simulink library "lib_fuel_cell2"  (Simulink 5.1)
values from neighbouring files (symbols this model uses):
  logFlag = 1    [advSACompMaskInit.m]    (also in advSACompMaskInitR13.m)
undefined symbols (not defined in the file or in its folder): fc_acc_mass, fc_base_mass, fc_c2i_th_cond, fc_c_init_tmp, fc_cl2h_eff, fc_co_map, fc_co_map_c2h, fc_cold, fc_cold_tmp, fc_cp, fc_eff_scale, fc_emisv, fc_exflow_map, fc_ext_sarea, fc_extmp_map, fc_fuel_den, fc_fuel_lhv, fc_fuel_map, fc_fuel_map_c2h, fc_h2x_th_cond, fc_h_air_flow, fc_h_cp, fc_hc_map, fc_hc_map_c2h, fc_hood_emisv, fc_hood_sarea, fc_i2x_th_cond, fc_i_init_tmp, fc_nox_map, fc_nox_map_c2h, fc_o2_map, fc_pm_map, fc_pm_map_c2h, fc_pwr_map, fc_pwr_scale, fc_tstat, pow
libraries: lib_etc x1
(part 2 of 2)

== system lib_fuel_cell2/fuel converter <fc> net model/Subsystem/Subsystem/fuel cell  system <fc>/Block NOTES ==
  note: 7/30/98
      | - started with battery from BD_SER2h.m
      | - added a Saturation block to prevent computed
      |        SOC from falling below 0 or rising above 1
      | - added logic in 'limit power' to prevent discharge
      | if SOC is below 0.001 (0.1%)
      | -added limit block to check if low SOC is preventing
      | discharge
  note: Power loss is computed as I*R+losses due to Coulombic (in)efficiency.
  note: This block models the energy storage system as an SOC-dependent voltage
      | in series with an SOC- and current direction-dependent internal resistance.
      | SOC is computed assuming that A-h capacity is a function of average discharge
      | current:  (A-h capacity)=ess_peukert_coeff * (average discharge current)^ess_peukert_exp.
      |
      | Discharge power is limited here so as not to bring the bus (battery pack) voltage below
      | the minimum controller voltage and so as to allow the solution of the quadratic eq'n for
      | discharge current.
      |
      | Positive current is discharge current in the convention used here.

== system lib_fuel_cell2/fuel converter <fc> net model/Subsystem/Subsystem/fuel cell  system <fc>/pwr vs. eff  fuel cell model ==
  net pwr req (W) : Inport
  Enable : EnablePort  StatesWhenEnabling=reset
  enforce limits : Subsystem
  net pwr avail (W) : Outport  OutputWhenDisabled=reset  InitialOutput=0
  wires:
  enforce limits/1(Out1) -> net pwr avail (W)/1
  net pwr req (W)/1 -> enforce limits/1(In1)

== system lib_fuel_cell2/fuel converter <fc> net model/Subsystem/Subsystem/fuel use and EO emis Fuel Cell/Block NOTES ==
  note: This block determines actual fuel use and engine-out emissions
      | given the fully hot values and the engine coolant temperature.
      | The correlations used here were developed at NREL using
      | FTP data collected under subcontract by JDM & Associates.
      | Note: PM hot/cold relation assumed same as HC

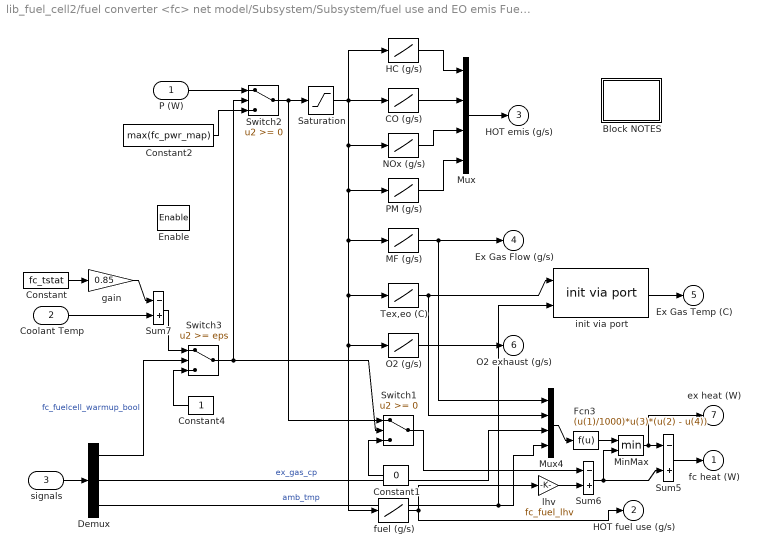
== system lib_fuel_cell2/fuel converter <fc> net model/Subsystem/Subsystem/fuel use and EO emis Fuel Cell/HOT engine maps  ==
  P (W) : Inport
  Coolant Temp : Inport  Port=2
  signals : Inport  Port=3
  Enable : EnablePort  StatesWhenEnabling=reset
  Block NOTES : Subsystem
      mask Display: disp('Block\nNOTES')
  CO (g/s) : Lookup  InputValues=fc_pwr_map*fc_pwr_scale  OutputValues=fc_co_map*fc_pwr_scale  SaturateOnIntegerOverflow=on
  Constant : Constant  Value=fc_tstat
  Constant1 : Constant  Orientation=left  Value=0
  Constant2 : Constant  Value=max(fc_pwr_map)
  Constant4 : Constant  Orientation=left
  Demux : Demux  Outputs=3
  Fcn3 : Fcn  Expr=(u(1)/1000)*u(3)*(u(2) - u(4))
  HC (g/s) : Lookup  InputValues=fc_pwr_map*fc_pwr_scale  OutputValues=fc_hc_map*fc_pwr_scale  SaturateOnIntegerOverflow=on
  MF (g/s) : Lookup  InputValues=fc_pwr_map*fc_pwr_scale  OutputValues=fc_exflow_map*fc_pwr_scale  SaturateOnIntegerOverflow=on
  MinMax : MinMax  Inputs=2
  Mux : Mux
  Mux4 : Mux
  NOx (g/s) : Lookup  InputValues=fc_pwr_map*fc_pwr_scale  OutputValues=fc_nox_map*fc_pwr_scale  SaturateOnIntegerOverflow=on
  O2 (g/s) : Lookup  InputValues=fc_pwr_map*fc_pwr_scale  OutputValues=fc_o2_map*fc_pwr_scale  SaturateOnIntegerOverflow=on
  PM (g/s) : Lookup  InputValues=fc_pwr_map*fc_pwr_scale  OutputValues=fc_pm_map*fc_pwr_scale  SaturateOnIntegerOverflow=on
  Saturation : Saturate  UpperLimit=max(fc_pwr_map*fc_pwr_scale)  LowerLimit=0
  Sum5 : Sum  Inputs=-+  SaturateOnIntegerOverflow=on  InputSameDT=on
  Sum6 : Sum  Inputs=-+  SaturateOnIntegerOverflow=on  InputSameDT=on
  Sum7 : Sum  Inputs=-+  SaturateOnIntegerOverflow=on  InputSameDT=on
  Switch1 : Switch  SaturateOnIntegerOverflow=on  InputSameDT=on
  Switch2 : Switch  SaturateOnIntegerOverflow=on  InputSameDT=on
  Switch3 : Switch  Threshold=eps  SaturateOnIntegerOverflow=on  InputSameDT=on
  Tex,eo (C) : Lookup  InputValues=fc_pwr_map*fc_pwr_scale  OutputValues=fc_extmp_map  SaturateOnIntegerOverflow=on
  fuel (g/s) : Lookup  InputValues=fc_pwr_map*fc_pwr_scale  OutputValues=fc_fuel_map*fc_pwr_scale/fc_eff_scale  SaturateOnIntegerOverflow=on
  gain : Gain  Gain=0.85  SaturateOnIntegerOverflow=on
  init via port : lib_etc/init via port  SimViewingDevice=off  DataTypeOverride=UseLocalSettings  MinMaxOverflowLogging=UseLocalSettings
      settings: Permissions=ReadWrite  RTWFcnNameOpts=Auto  RTWFileNameOpts=Auto
  lhv : Gain  Gain=fc_fuel_lhv  SaturateOnIntegerOverflow=on
  fc heat (W) : Outport  OutputWhenDisabled=reset  InitialOutput=eps
  HOT fuel use (g/s) : Outport  Port=2  OutputWhenDisabled=reset  InitialOutput=eps
  HOT emis (g/s) : Outport  Port=3  OutputWhenDisabled=reset  InitialOutput=eps
  Ex Gas Flow (g/s) : Outport  Port=4  OutputWhenDisabled=reset  InitialOutput=eps
  Ex Gas Temp (C) : Outport  Port=5
  O2 exhaust (g/s) : Outport  Port=6  OutputWhenDisabled=reset  InitialOutput=eps
  ex heat (W) : Outport  Port=7  OutputWhenDisabled=reset  InitialOutput=eps
  wires:
  O2 (g/s)/1 -> O2 exhaust (g/s)/1
  fuel (g/s)/1 -> HOT fuel use (g/s)/1, lhv/1
  Constant1/1 -> Switch1/3
  lhv/1 -> Sum6/2
  Sum6/1 -> MinMax/2, Sum5/2
  MinMax/1 -> ex heat (W)/1, Sum5/1
  Fcn3/1 -> MinMax/1
  Sum5/1 -> fc heat (W)/1
  Mux4/1 -> Fcn3/1
  Switch1/1 -> Sum6/1
  CO (g/s)/1 -> Mux/2
  Saturation/1 -> HC (g/s)/1, NOx (g/s)/1, PM (g/s)/1, O2 (g/s)/1, fuel (g/s)/1, Tex,eo (C)/1, MF (g/s)/1, CO (g/s)/1
  Tex,eo (C)/1 -> Mux4/2, init via port/1
  MF (g/s)/1 -> Mux4/1, Ex Gas Flow (g/s)/1
  Mux/1 -> HOT emis (g/s)/1
  NOx (g/s)/1 -> Mux/3
  HC (g/s)/1 -> Mux/1
  PM (g/s)/1 -> Mux/4
  P (W)/1 -> Switch2/1
  Constant2/1 -> Switch2/3
  Switch2/1 -> Saturation/1, Switch1/1
  Switch3/1 -> Switch1/2, Switch2/2
  Sum7/1 -> Switch3/1
  gain/1 -> Sum7/1
  Coolant Temp/1 -> Sum7/2
  Constant/1 -> gain/1
  Constant4/1 -> Switch3/3
  Demux/2 -> Mux4/3  "ex_gas_cp"
  Demux/3 -> Mux4/4, init via port/2  "amb_tmp"
  init via port/1 -> Ex Gas Temp (C)/1
  signals/1 -> Demux/1
  Demux/1 -> Switch3/2  "fc_fuelcell_warmup_bool"

== system lib_fuel_cell2/fuel converter <fc> net model/Subsystem/Subsystem/fuel use and EO emis Fuel Cell/System  Efficiency ==
  In1 : Inport
  Constant : Constant  Value=eps
  Gain : Gain  Gain=fc_fuel_lhv  SaturateOnIntegerOverflow=on
  Gain1 : Gain  Gain=100  SaturateOnIntegerOverflow=on
  Product : Product  Inputs=*/  SaturateOnIntegerOverflow=on  InputSameDT=on
  Sum1 : Sum  Inputs=|++  SaturateOnIntegerOverflow=on  InputSameDT=on
  enhancedToWorkspace : Subsystem  TreatAsAtomicUnit=on  mask(enhancedToWorkspace){generalName=generalName, specificName=eff_out_a, logFlag=logFlag}
      mask prompts: generalName "General Name [char-evaluated]"; specificName "Specific Name [char-literal]"; logFlag "Enable flag (1=on,0=off)"
      mask help: A wrapper for the Simulink "To Workspace" block that allows you to evaluate the name of the variable to log to workspace. This is useful to avoid the double logging errors that occur when you pull in two library models that attempt to log to the same variable.
      mask init:
      | enhancedToWsMaker
      settings: CopyFcn=breakLinkCopyFcn  ParentCloseFcn=breakLinkParCloseFcn
      mask Help:
      | <h2>Enhanced To Workspace Block</h2>
      | <h3>Parameters</h3>
      | <UL>
      | <li><b>General Name:</b> This is the more general name of the variable. Variables are saved to the workspace as <i>generalName_specificName</i>. Note that this is an evaluated variable. If you would like to type in the value directly, it must be surrounded with single quotes. Otherwise you can input the name of a variable containing a char string.</li>
      | <li><b>Specific Name:</b> This is the specific name of the variable. Note that this is input as a char literal (i.e., you don't need quotes).</li>
      | <li><b>Enable Flag:</b> This flag should have the value of 0 or 1. If 0, the variable will not be logged to the workspace. If 1, the variable will be logged. This is done so that variable logging can be turned off to improve speed.</li>
      | </ul>
      | <h3>Overview</h3>
      | <p>The enhanced to workspace block was put together to allow one to dynamically resolve variable names at run time in simulink. This is most powerful when used in conjunction with a masked subsystem to allow multiple instances of that masked subsytem to be used in the same model. The strategy is to set the generalName in the block mask which will allow the block to change the general name for all variable logging on the fly.
      | <h3>Helper Files</h3>
      | <p>Three m-files are required by the enhancedToWorkspace block. These files are located in the &lt; ADVISOR root &gt;/GUI directory :
      | <ul>
      | <li><i>enhancedToWsMaker.m</i> This file runs the mask initialization for the block</li>
      | <li><i>breakLinkCopyFcn.m</i> This file is used by the block callback when the simulink block is copied. It is necessary to break the link to the enhancedToWorkspace similar to the To Workspace block in order for it to be able to configure itself. (Try copying simulink's To Workspace block--it is impossible to make a link)</li>
      | <li><i>breakLinkParCloseFcn.m</i> This file is similar to the breakLinkCopyFcn and is used when a parent system is closed</li>
      | </ul>
      | <hr>
      | 
      | <p>Created 2003-Jan-21, Michael Patrick O'Keefe, NREL</p>
      | 
      | <!--
      | <VARDEF>
      | <H3>var_name</H3>
      | <UL>
      | <LI><B>data type</B> data type here</LI>
      | <LI><B>units</B> units here</LI>
      | <LI><B>vehicle type</B> vehicle type here</LI>
      | <LI><B>description</B> description here</LI>
      | </UL>
      | </VARDEF>
      | -->
      mask Display: disp([generalName,'_',specificName])
  tag scope: fc_eff_out_a=scoped
  wires:
  [fc_pwr_out_a] -> Product/1
  Product/1 -> Gain1/1
  Gain/1 -> Sum1/1
  Constant/1 -> Sum1/2
  Sum1/1 -> Product/2
  Gain1/1 -> [fc_eff_out_a], enhancedToWorkspace/1(In1)
  In1/1 -> Gain/1

== system lib_fuel_cell2/fuel converter <fc> net model/Subsystem/Subsystem/fuel use and EO emis Fuel Cell/enhancedToWorkspace ==
  In1 : Inport
  To Workspace : ToWorkspace  VariableName=fuel_cell__ex_th_pwr  SampleTime=-1  SaveFormat=Array
  wires:
  In1/1 -> To Workspace/1

== system lib_fuel_cell2/fuel converter <fc> net model/Subsystem/Subsystem/fuel use and EO emis Fuel Cell/enhancedToWorkspace1 ==
  In1 : Inport
  To Workspace : ToWorkspace  VariableName=fuel_cell__o2_flow  SampleTime=-1  SaveFormat=Array
  wires:
  In1/1 -> To Workspace/1

== system lib_fuel_cell2/fuel converter <fc> net model/Subsystem/Subsystem/fuel use and EO emis Fuel Cell/enhancedToWorkspace10 ==
  In1 : Inport
  To Workspace : ToWorkspace  VariableName=fuel_cell__r_th_pwr  SampleTime=-1  SaveFormat=Array
  wires:
  In1/1 -> To Workspace/1

== system lib_fuel_cell2/fuel converter <fc> net model/Subsystem/Subsystem/fuel use and EO emis Fuel Cell/enhancedToWorkspace2 ==
  In1 : Inport
  To Workspace : ToWorkspace  VariableName=fuel_cell__ex_gas_tmp  SampleTime=-1  SaveFormat=Array
  wires:
  In1/1 -> To Workspace/1

== system lib_fuel_cell2/fuel converter <fc> net model/Subsystem/Subsystem/fuel use and EO emis Fuel Cell/enhancedToWorkspace3 ==
  In1 : Inport
  To Workspace : ToWorkspace  VariableName=fuel_cell__ex_gas_flow  SampleTime=-1  SaveFormat=Array
  wires:
  In1/1 -> To Workspace/1

== system lib_fuel_cell2/fuel converter <fc> net model/Subsystem/Subsystem/fuel use and EO emis Fuel Cell/enhancedToWorkspace4 ==
  In1 : Inport
  To Workspace : ToWorkspace  VariableName=fuel_cell__emis_eo  SampleTime=-1  SaveFormat=Array
  wires:
  In1/1 -> To Workspace/1

== system lib_fuel_cell2/fuel converter <fc> net model/Subsystem/Subsystem/fuel use and EO emis Fuel Cell/enhancedToWorkspace5 ==
  In1 : Inport
  To Workspace : ToWorkspace  VariableName=fuel_cell__fuel_rate  SampleTime=-1  SaveFormat=Array
  wires:
  In1/1 -> To Workspace/1

== system lib_fuel_cell2/fuel converter <fc> net model/Subsystem/Subsystem/fuel use and EO emis Fuel Cell/enhancedToWorkspace6 ==
  In1 : Inport
  To Workspace : ToWorkspace  VariableName=fuel_cell__th_pwr  SampleTime=-1  SaveFormat=Array
  wires:
  In1/1 -> To Workspace/1

== system lib_fuel_cell2/fuel converter <fc> net model/Subsystem/Subsystem/fuel use and EO emis Fuel Cell/enhancedToWorkspace7 ==
  In1 : Inport
  To Workspace : ToWorkspace  VariableName=fuel_cell__clt_tmp  SampleTime=-1  SaveFormat=Array
  wires:
  In1/1 -> To Workspace/1

== system lib_fuel_cell2/fuel converter <fc> net model/Subsystem/Subsystem/fuel use and EO emis Fuel Cell/enhancedToWorkspace8 ==
  In1 : Inport
  To Workspace : ToWorkspace  VariableName=fuel_cell__tmp  SampleTime=-1  SaveFormat=Array
  wires:
  In1/1 -> To Workspace/1

== system lib_fuel_cell2/fuel converter <fc> net model/Subsystem/Subsystem/fuel use and EO emis Fuel Cell/enhancedToWorkspace9 ==
  In1 : Inport
  To Workspace : ToWorkspace  VariableName=fuel_cell__h_th_pwr  SampleTime=-1  SaveFormat=Array
  wires:
  In1/1 -> To Workspace/1

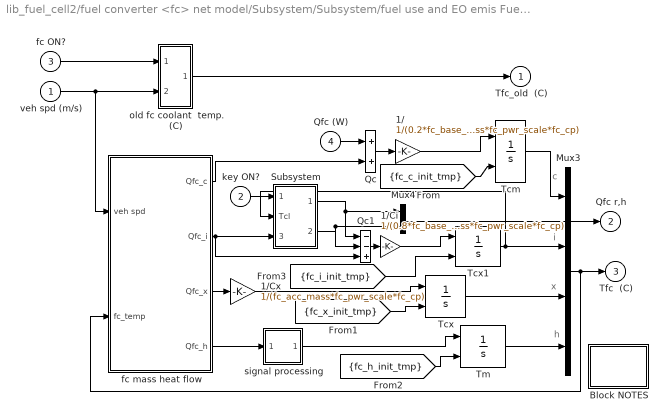
== system lib_fuel_cell2/fuel converter <fc> net model/Subsystem/Subsystem/fuel use and EO emis Fuel Cell/fc temp ==
  note: c
  note: i
  note: x
  note: h
  veh spd (m/s) : Inport
  key ON? : Inport  Port=2
  fc ON? : Inport  Port=3
  Qfc (W) : Inport  Port=4
  1/ : Gain  Gain=1/(0.2*fc_base_mass*fc_pwr_scale*fc_cp)  SaturateOnIntegerOverflow=on
  1/Ci : Gain  Gain=1/(0.8*fc_base_mass*fc_pwr_scale*fc_cp)  SaturateOnIntegerOverflow=on
  1/Cx : Gain  Gain=1/(fc_acc_mass*fc_pwr_scale*fc_cp)  SaturateOnIntegerOverflow=on
  Block NOTES : Subsystem
      mask Display: disp('Block\nNOTES')
  Mux3 : Mux
  Mux4 : Mux  Inputs=2
  Qc : Sum  SaturateOnIntegerOverflow=on  InputSameDT=on
  Qc1 : Sum  Inputs=--+  SaturateOnIntegerOverflow=on  InputSameDT=on
  Subsystem : Subsystem
  Tcm : Integrator  InitialConditionSource=external  InitialCondition=fc_c_init_tmp
  Tcx : Integrator  InitialConditionSource=external
  Tcx1 : Integrator  InitialConditionSource=external
  Tm : Integrator  InitialConditionSource=external
  fc mass heat flow : Subsystem
  old fc coolant  temp. (C) : Subsystem
  signal processing : Subsystem
  Tfc_old  (C) : Outport  InitialOutput=0
  Qfc r,h : Outport  Port=2  InitialOutput=0
  Tfc  (C) : Outport  Port=3  InitialOutput=0
  wires:
  fc ON?/1 -> old fc coolant  temp. (C)/1(fc on?)
  veh spd (m/s)/1 -> fc mass heat flow/1(veh spd), old fc coolant  temp. (C)/2(veh spd)
  old fc coolant  temp. (C)/1(fc coolant  temp (C)) -> Tfc_old  (C)/1
  Mux3/1 -> Tfc  (C)/1, fc mass heat flow/2(fc_temp)
  fc mass heat flow/4(Qfc_h) -> signal processing/1(In1)
  signal processing/1(Out1) -> Tm/1
  Tm/1 -> Mux3/4
  Tcx/1 -> Mux3/3
  key ON?/1 -> Subsystem/1(In1)
  fc mass heat flow/3(Qfc_x) -> 1/Cx/1
  1/Cx/1 -> Tcx/1
  Mux4/1 -> Qfc r,h/1
  Tcx1/1 -> Mux3/2, Subsystem/2(Tcl)
  Subsystem/1(Out1) -> Mux4/1, Qc1/1
  Subsystem/2(Out2) -> Mux4/2, Qc1/2
  fc mass heat flow/2(Qfc_i) -> Qc1/3, Subsystem/3(Qfc_i)
  Tcm/1 -> Mux3/1
  1/Ci/1 -> Tcx1/1
  Qc1/1 -> 1/Ci/1
  fc mass heat flow/1(Qfc_c) -> Qc/2
  Qfc (W)/1 -> Qc/1
  1//1 -> Tcm/1
  Qc/1 -> 1//1
  [fc_c_init_tmp] -> Tcm/2
  [fc_x_init_tmp] -> Tcx/2
  [fc_h_init_tmp] -> Tm/2
  [fc_i_init_tmp] -> Tcx1/2

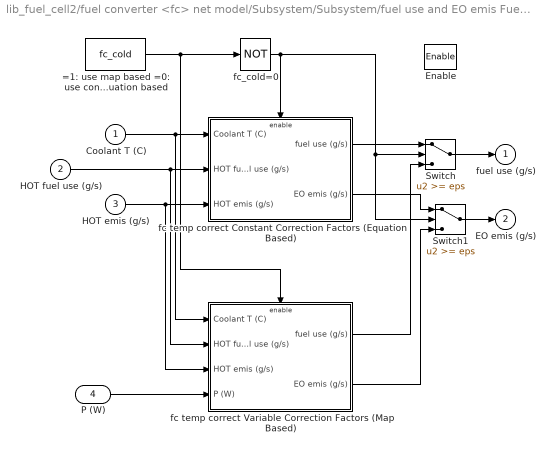
== system lib_fuel_cell2/fuel converter <fc> net model/Subsystem/Subsystem/fuel use and EO emis Fuel Cell/fc temp correct ==
  Coolant T (C) : Inport
  HOT fuel use (g/s) : Inport  Port=2
  HOT emis (g/s) : Inport  Port=3
  P (W) : Inport  Port=4
  Enable : EnablePort  StatesWhenEnabling=reset
  =1: use map based =0: use constant equation based : Constant  Value=fc_cold
  Switch : Switch  Threshold=eps  SaturateOnIntegerOverflow=on  InputSameDT=on
  Switch1 : Switch  Threshold=eps  SaturateOnIntegerOverflow=on  InputSameDT=on
  fc temp correct Constant Correction Factors (Equation Based) : Subsystem  TreatAsAtomicUnit=on
  fc temp correct Variable Correction Factors (Map Based) : Subsystem  TreatAsAtomicUnit=on
  fc_cold=0 : Logic  Operator=NOT
  fuel use (g/s) : Outport  OutputWhenDisabled=reset  InitialOutput=0
  EO emis (g/s) : Outport  Port=2  OutputWhenDisabled=reset  InitialOutput=0
  wires:
  P (W)/1 -> fc temp correct Variable Correction Factors (Map Based)/4(P (W))
  =1: use map based =0: use constant equation based/1 -> fc_cold=0/1, fc temp correct Variable Correction Factors (Map Based)/Enable
  Coolant T (C)/1 -> fc temp correct Constant Correction Factors (Equation Based)/1(Coolant T (C)), fc temp correct Variable Correction Factors (Map Based)/1(Coolant T (C))
  HOT fuel use (g/s)/1 -> fc temp correct Constant Correction Factors (Equation Based)/2(HOT fuel use (g/s)), fc temp correct Variable Correction Factors (Map Based)/2(HOT fuel use (g/s))
  HOT emis (g/s)/1 -> fc temp correct Constant Correction Factors (Equation Based)/3(HOT emis (g/s)), fc temp correct Variable Correction Factors (Map Based)/3(HOT emis (g/s))
  fc temp correct Constant Correction Factors (Equation Based)/1(fuel use (g/s)) -> Switch/1
  fc_cold=0/1 -> fc temp correct Constant Correction Factors (Equation Based)/Enable, Switch/2, Switch1/2
  fc temp correct Variable Correction Factors (Map Based)/1(fuel use (g/s)) -> Switch/3
  fc temp correct Constant Correction Factors (Equation Based)/2(EO emis (g/s)) -> Switch1/1
  fc temp correct Variable Correction Factors (Map Based)/2(EO emis (g/s)) -> Switch1/3
  Switch/1 -> fuel use (g/s)/1
  Switch1/1 -> EO emis (g/s)/1

== system lib_fuel_cell2/fuel converter <fc> net model/Subsystem/Subsystem/fuel cell  system <fc>/pwr vs. eff  fuel cell model/enforce limits ==
  In1 : Inport
  Saturation : Saturate  UpperLimit=max(fc_pwr_map)*fc_pwr_scale  LowerLimit=0
  Out1 : Outport  InitialOutput=0
  wires:
  In1/1 -> Saturation/1
  Saturation/1 -> Out1/1

== system lib_fuel_cell2/fuel converter <fc> net model/Subsystem/Subsystem/fuel use and EO emis Fuel Cell/HOT engine maps /Block NOTES ==
  note: This block determines the fully hot fuel use, engine-out emissions output rates, exhaust gas mass flow rate,
      | and engine-out exhaust gas temperature as a function of engine output torque and speed.
      | The engine maps (except for exhaust gas temperature) can be scaled using variables fc_spd_scale and
      |  fc_trq_scale; it is recommended that scaling values outside the range of 0.85 to 1.15 be used CAREFULLY.

== system lib_fuel_cell2/fuel converter <fc> net model/Subsystem/Subsystem/fuel use and EO emis Fuel Cell/System  Efficiency/enhancedToWorkspace ==
  In1 : Inport
  To Workspace : ToWorkspace  VariableName=fuel_cell__eff_out_a  SampleTime=-1  SaveFormat=Array
  wires:
  In1/1 -> To Workspace/1

== system lib_fuel_cell2/fuel converter <fc> net model/Subsystem/Subsystem/fuel use and EO emis Fuel Cell/fc temp/Block NOTES ==
  note: This block models the thermal behavior internal combustion engine (ICE).
      | Emphasis is on the coolant since this temperature is used to correct engine
      | fuel use.

== system lib_fuel_cell2/fuel converter <fc> net model/Subsystem/Subsystem/fuel use and EO emis Fuel Cell/fc temp/Subsystem ==
  In1 : Inport  Orientation=down
  Tcl : Inport  Port=2
  Qfc_i : Inport  Port=3
  fc coolant : Subsystem  TreatAsAtomicUnit=on
  Out1 : Outport
  Out2 : Outport  Port=2
  wires:
  Tcl/1 -> fc coolant/1(Tcl)
  Qfc_i/1 -> fc coolant/2("Qfc_i ")
  In1/1 -> fc coolant/Enable
  fc coolant/1(Qfc_rad) -> Out1/1
  fc coolant/2(Qfc_htr) -> Out2/1
  [amb_tmp] -> fc coolant/3(amb_tmp)
  [air_cp] -> fc coolant/4(air_cp)

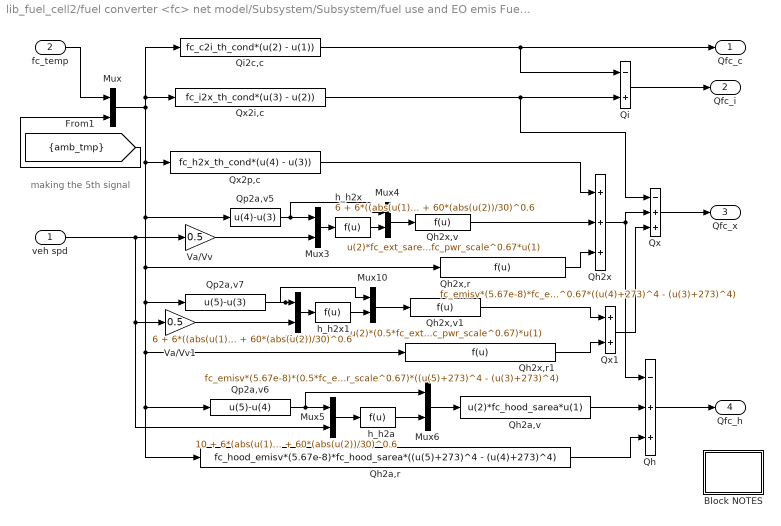
== system lib_fuel_cell2/fuel converter <fc> net model/Subsystem/Subsystem/fuel use and EO emis Fuel Cell/fc temp/fc mass heat flow ==
  note: making the 5th signal
  veh spd : Inport
  fc_temp : Inport  Port=2
  Block NOTES : Subsystem
      mask Display: disp('Block\nNOTES')
  Mux{,3..6,9..10} (7 alike) : Mux  Inputs=2
  Qh : Sum  Inputs=-++  SaturateOnIntegerOverflow=on  InputSameDT=on
  Qh2a,r : Fcn  Expr=fc_hood_emisv*(5.67e-8)*fc_hood_sarea*((u(5)+273)^4 - (u(4)+273)^4)
  Qh2a,v : Fcn  Expr=u(2)*fc_hood_sarea*u(1)
  Qh2x : Sum  Inputs=+++  SaturateOnIntegerOverflow=on  InputSameDT=on
  Qh2x,r : Fcn  Expr=fc_emisv*(5.67e-8)*fc_ext_sarea*fc_pwr_scale^0.67*((u(4)+273)^4 - (u(3)+273)^4)
  Qh2x,r1 : Fcn  Expr=fc_emisv*(5.67e-8)*(0.5*fc_ext_sarea*fc_pwr_scale^0.67)*((u(5)+273)^4 - (u(3)+273)^4)
  Qh2x,v : Fcn  Expr=u(2)*fc_ext_sarea*fc_pwr_scale^0.67*u(1)
  Qh2x,v1 : Fcn  Expr=u(2)*(0.5*fc_ext_sarea*fc_pwr_scale^0.67)*u(1)
  Qi : Sum  Inputs=-+  SaturateOnIntegerOverflow=on  InputSameDT=on
  Qi2c,c : Fcn  Expr=fc_c2i_th_cond*(u(2) - u(1))
  Qp2a,v5 : Fcn  Expr=u(4)-u(3)
  Qp2a,v6 : Fcn  Expr=u(5)-u(4)
  Qp2a,v7 : Fcn  Expr=u(5)-u(3)
  Qx : Sum  Inputs=-++  SaturateOnIntegerOverflow=on  InputSameDT=on
  Qx1 : Sum  SaturateOnIntegerOverflow=on  InputSameDT=on
  Qx2i,c : Fcn  Expr=fc_i2x_th_cond*(u(3) - u(2))
  Qx2p,c : Fcn  Expr=fc_h2x_th_cond*(u(4) - u(3))
  Va/Vv : Gain  Gain=0.5  SaturateOnIntegerOverflow=on
  Va/Vv1 : Gain  Gain=0.5  SaturateOnIntegerOverflow=on
  h_h2a : Fcn  Expr=10 + 6*(abs(u(1))/1000)^0.3 + 60*(abs(u(2))/30)^0.6
  h_h2x : Fcn  Expr=6 + 6*((abs(u(1))/1000))^0.3 + 60*(abs(u(2))/30)^0.6
  h_h2x1 : Fcn  Expr=6 + 6*((abs(u(1))/1000))^0.3 + 60*(abs(u(2))/30)^0.6
  Qfc_c : Outport
  Qfc_i : Outport  Port=2
  Qfc_x : Outport  Port=3
  Qfc_h : Outport  Port=4
  wires:
  Mux10/1 -> Qh2x,v1/1
  Mux9/1 -> h_h2x1/1
  Qp2a,v7/1 -> Mux9/1, Mux10/1
  h_h2x1/1 -> Mux10/2
  Va/Vv1/1 -> Mux9/2
  Mux4/1 -> Qh2x,v/1
  Mux3/1 -> h_h2x/1
  Qp2a,v5/1 -> Mux3/1, Mux4/1
  h_h2x/1 -> Mux4/2
  veh spd/1 -> Va/Vv/1, Mux5/2, Va/Vv1/1
  Va/Vv/1 -> Mux3/2
  Qi2c,c/1 -> Qfc_c/1, Qi/1
  fc_temp/1 -> Mux/1
  Qx2i,c/1 -> Qi/2, Qx/1
  Qi/1 -> Qfc_i/1
  Qx/1 -> Qfc_x/1
  Qh2x/1 -> Qx/2, Qh/1
  Qh/1 -> Qfc_h/1
  Mux6/1 -> Qh2a,v/1
  Mux5/1 -> h_h2a/1
  Qp2a,v6/1 -> Mux5/1, Mux6/1
  h_h2a/1 -> Mux6/2
  Qx1/1 -> Qx/3
  Qh2x,v/1 -> Qh2x/2
  Qx2p,c/1 -> Qh2x/1
  Qh2x,r1/1 -> Qx1/2
  Qh2x,v1/1 -> Qx1/1
  Qh2a,r/1 -> Qh/3
  Qh2a,v/1 -> Qh/2
  Qh2x,r/1 -> Qh2x/3
  [amb_tmp] -> Mux/2
  Mux/1 -> Qi2c,c/1, Qx2i,c/1, Qx2p,c/1, Qp2a,v7/1, Qp2a,v6/1, Qh2a,r/1, Qh2x,r1/1, Qh2x,r/1, Qp2a,v5/1

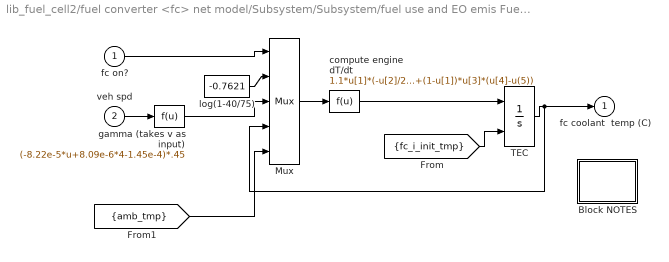
== system lib_fuel_cell2/fuel converter <fc> net model/Subsystem/Subsystem/fuel use and EO emis Fuel Cell/fc temp/old fc coolant  temp. (C) ==
  fc on? : Inport
  veh spd : Inport  Port=2
  Block NOTES : Subsystem
      mask Display: disp('Block\nNOTES')
  Mux : Mux  Inputs=5
  TEC : Integrator  InitialConditionSource=external  InitialCondition=fc_i_init_tmp
  compute engine dT/dt : Fcn  Expr=1.1*u[1]*(-u[2]/218)*(95-u[4])+(1-u[1])*u[3]*(u[4]-u(5))
  gamma (takes v as input) : Fcn  Expr=(-8.22e-5*u+8.09e-6*4-1.45e-4)*.45
  log(1-40/75) : Constant  Value=-0.7621
  fc coolant  temp (C) : Outport  InitialOutput=0
  wires:
  compute engine dT/dt/1 -> TEC/1
  gamma (takes v as input)/1 -> Mux/3
  log(1-40/75)/1 -> Mux/2
  Mux/1 -> compute engine dT/dt/1
  fc on?/1 -> Mux/1
  veh spd/1 -> gamma (takes v as input)/1
  TEC/1 -> fc coolant  temp (C)/1, Mux/4
  [fc_i_init_tmp] -> TEC/2
  [amb_tmp] -> Mux/5

== system lib_fuel_cell2/fuel converter <fc> net model/Subsystem/Subsystem/fuel use and EO emis Fuel Cell/fc temp/signal processing ==
  note: 1/(0.1*veh_glider_mass*fc_pwr_scale*fc_h_cp)
  In1 : Inport
  Constant : Constant  Value=0.1
  Product : Product  Inputs=*////  SaturateOnIntegerOverflow=on
  Out1 : Outport
  wires:
  Constant/1 -> Product/2
  [veh_glider_mass] -> Product/3
  [fc_pwr_scale] -> Product/4
  [fc_h_cp] -> Product/5
  In1/1 -> Product/1
  Product/1 -> Out1/1

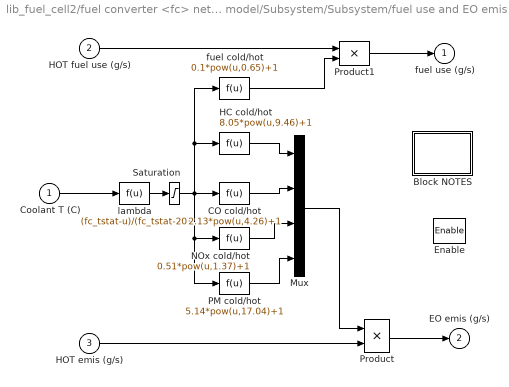
== system lib_fuel_cell2/fuel converter <fc> net model/Subsystem/Subsystem/fuel use and EO emis Fuel Cell/fc temp correct/fc temp correct Constant Correction Factors (Equation Based) ==
  Coolant T (C) : Inport
  HOT fuel use (g/s) : Inport  Port=2
  HOT emis (g/s) : Inport  Port=3
  Enable : EnablePort  StatesWhenEnabling=reset
  Block NOTES : Subsystem
      mask Display: disp('Block\nNOTES')
  CO cold/hot : Fcn  Expr=2.13*pow(u,4.26)+1
  HC cold/hot : Fcn  Expr=8.05*pow(u,9.46)+1
  Mux : Mux
  NOx cold/hot : Fcn  Expr=0.51*pow(u,1.37)+1
  PM cold/hot : Fcn  Expr=5.14*pow(u,17.04)+1
  Product : Product  SaturateOnIntegerOverflow=on  InputSameDT=on
  Product1 : Product  SaturateOnIntegerOverflow=on  InputSameDT=on
  Saturation : Saturate  UpperLimit=1  LowerLimit=0
  fuel cold/hot : Fcn  Expr=0.1*pow(u,0.65)+1
  lambda : Fcn  Expr=(fc_tstat-u)/(fc_tstat-20)
  fuel use (g/s) : Outport  OutputWhenDisabled=reset  InitialOutput=0
  EO emis (g/s) : Outport  Port=2  OutputWhenDisabled=reset  InitialOutput=0
  wires:
  HOT emis (g/s)/1 -> Product/2
  Coolant T (C)/1 -> lambda/1
  HOT fuel use (g/s)/1 -> Product1/1
  Product1/1 -> fuel use (g/s)/1
  CO cold/hot/1 -> Mux/2
  Product/1 -> EO emis (g/s)/1
  fuel cold/hot/1 -> Product1/2
  Mux/1 -> Product/1
  lambda/1 -> Saturation/1
  Saturation/1 -> PM cold/hot/1, NOx cold/hot/1, fuel cold/hot/1, HC cold/hot/1, CO cold/hot/1
  HC cold/hot/1 -> Mux/1
  NOx cold/hot/1 -> Mux/3
  PM cold/hot/1 -> Mux/4

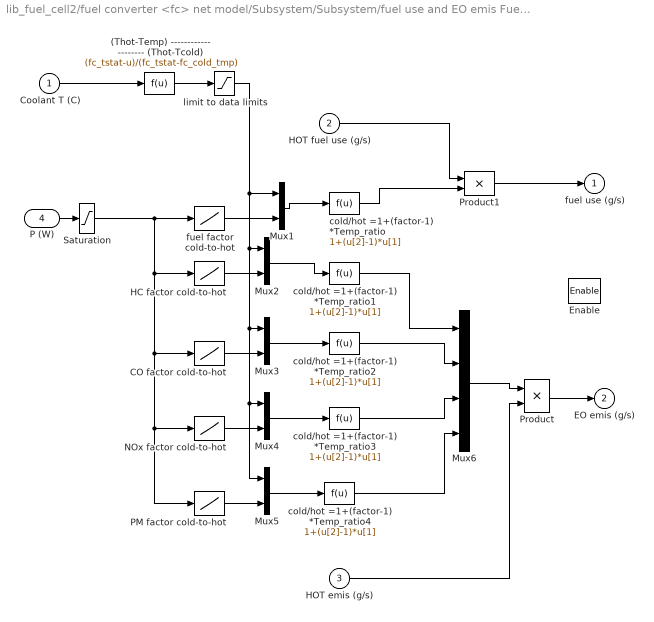
== system lib_fuel_cell2/fuel converter <fc> net model/Subsystem/Subsystem/fuel use and EO emis Fuel Cell/fc temp correct/fc temp correct Variable Correction Factors (Map Based) ==
  Coolant T (C) : Inport
  HOT fuel use (g/s) : Inport  Port=2
  HOT emis (g/s) : Inport  Port=3
  P (W) : Inport  Port=4
  Enable : EnablePort  StatesWhenEnabling=reset
  (Thot-Temp) -------------------- (Thot-Tcold) : Fcn  Expr=(fc_tstat-u)/(fc_tstat-fc_cold_tmp)
  CO factor cold-to-hot : Lookup  InputValues=fc_pwr_map*fc_pwr_scale  OutputValues=fc_co_map_c2h  SaturateOnIntegerOverflow=on
  HC factor cold-to-hot : Lookup  InputValues=fc_pwr_map*fc_pwr_scale  OutputValues=fc_hc_map_c2h  SaturateOnIntegerOverflow=on
  Mux{1..5} (5 alike) : Mux  Inputs=2
  Mux6 : Mux
  NOx factor cold-to-hot : Lookup  InputValues=fc_pwr_map*fc_pwr_scale  OutputValues=fc_nox_map_c2h  SaturateOnIntegerOverflow=on
  PM factor cold-to-hot : Lookup  InputValues=fc_pwr_map*fc_pwr_scale  OutputValues=fc_pm_map_c2h  SaturateOnIntegerOverflow=on
  Product : Product  SaturateOnIntegerOverflow=on  InputSameDT=on
  Product1 : Product  SaturateOnIntegerOverflow=on  InputSameDT=on
  Saturation : Saturate  UpperLimit=max(fc_pwr_map*fc_pwr_scale)  LowerLimit=0
  cold/hot =1+(factor-1) *Temp_ratio{,1..4} (5 alike) : Fcn  Expr=1+(u[2]-1)*u[1]
  fuel factor cold-to-hot : Lookup  InputValues=fc_pwr_map*fc_pwr_scale  OutputValues=fc_fuel_map_c2h  SaturateOnIntegerOverflow=on
  limit to data limits : Saturate  UpperLimit=1  LowerLimit=0
  fuel use (g/s) : Outport  OutputWhenDisabled=reset  InitialOutput=0
  EO emis (g/s) : Outport  Port=2  OutputWhenDisabled=reset  InitialOutput=0
  wires:
  cold/hot =1+(factor-1) *Temp_ratio4/1 -> Mux6/4
  cold/hot =1+(factor-1) *Temp_ratio3/1 -> Mux6/3
  cold/hot =1+(factor-1) *Temp_ratio2/1 -> Mux6/2
  cold/hot =1+(factor-1) *Temp_ratio1/1 -> Mux6/1
  cold/hot =1+(factor-1) *Temp_ratio/1 -> Product1/2
  limit to data limits/1 -> Mux1/1, Mux2/1, Mux3/1, Mux4/1, Mux5/1
  (Thot-Temp) -------------------- (Thot-Tcold)/1 -> limit to data limits/1
  Saturation/1 -> PM factor cold-to-hot/1, NOx factor cold-to-hot/1, CO factor cold-to-hot/1, HC factor cold-to-hot/1, fuel factor cold-to-hot/1
  P (W)/1 -> Saturation/1
  HOT fuel use (g/s)/1 -> Product1/1
  Coolant T (C)/1 -> (Thot-Temp) -------------------- (Thot-Tcold)/1
  fuel factor cold-to-hot/1 -> Mux1/2
  Mux1/1 -> cold/hot =1+(factor-1) *Temp_ratio/1
  HC factor cold-to-hot/1 -> Mux2/2
  CO factor cold-to-hot/1 -> Mux3/2
  NOx factor cold-to-hot/1 -> Mux4/2
  PM factor cold-to-hot/1 -> Mux5/2
  Mux2/1 -> cold/hot =1+(factor-1) *Temp_ratio1/1
  Mux3/1 -> cold/hot =1+(factor-1) *Temp_ratio2/1
  Mux4/1 -> cold/hot =1+(factor-1) *Temp_ratio3/1
  Mux5/1 -> cold/hot =1+(factor-1) *Temp_ratio4/1
  Product1/1 -> fuel use (g/s)/1
  Product/1 -> EO emis (g/s)/1
  HOT emis (g/s)/1 -> Product/2
  Mux6/1 -> Product/1

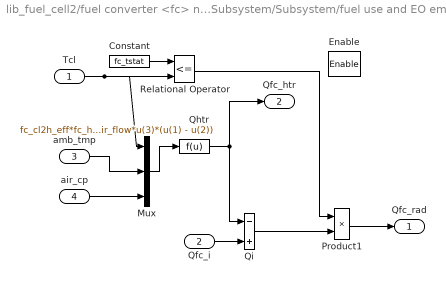
== system lib_fuel_cell2/fuel converter <fc> net model/Subsystem/Subsystem/fuel use and EO emis Fuel Cell/fc temp/Subsystem/fc coolant ==
  Tcl : Inport
  "Qfc_i " : Inport  Port=2
  amb_tmp : Inport  Port=3
  air_cp : Inport  Port=4
  Enable : EnablePort  StatesWhenEnabling=reset
  Constant : Constant  Value=fc_tstat
  Mux : Mux  Inputs=3
  Product1 : Product  SaturateOnIntegerOverflow=on  InputSameDT=on
  Qhtr : Fcn  Expr=fc_cl2h_eff*fc_h_air_flow*u(3)*(u(1) - u(2))
  Qi : Sum  Inputs=-+  SaturateOnIntegerOverflow=on  InputSameDT=on
  Relational Operator : RelationalOperator  Operator=<=  InputSameDT=on
  Qfc_rad : Outport  OutputWhenDisabled=reset  InitialOutput=0
  Qfc_htr : Outport  Port=2  OutputWhenDisabled=reset  InitialOutput=0
  wires:
  Tcl/1 -> Relational Operator/2, Mux/1
  Relational Operator/1 -> Product1/1
  Constant/1 -> Relational Operator/1
  Product1/1 -> Qfc_rad/1
  "Qfc_i "/1 -> Qi/2
  Qhtr/1 -> Qi/1, Qfc_htr/1
  Qi/1 -> Product1/2
  Mux/1 -> Qhtr/1
  amb_tmp/1 -> Mux/2
  air_cp/1 -> Mux/3

== system lib_fuel_cell2/fuel converter <fc> net model/Subsystem/Subsystem/fuel use and EO emis Fuel Cell/fc temp/fc mass heat flow/Block NOTES ==
  note: FUEL CONVERTER MASS HEAT LOSS
      | This block models the heat loss from a fuel converter (such as an IC engine).
      | Convection (as a function of vehicle speed), radiation, and conduction effects are included.
      | Engine cylinder (c), interior (i), exterior (x) and hood (h)
      | heat flows are estimated based on the temperatures from the previous iteration.

== system lib_fuel_cell2/fuel converter <fc> net model/Subsystem/Subsystem/fuel use and EO emis Fuel Cell/fc temp/old fc coolant  temp. (C)/Block NOTES ==
  note: This block computes engine coolant temperature,
      | assuming that it asymptotically approaches its maximum
      | temperature when the engine is on, and asymptotically
      | approaches the ambient temperature when the engine
      | is off.  Temperatue rise rate is assumed to be a function
      | only of current engine coolant temperature, and the fall
      | rate is also a function of vehicle speed and ambient temperature.
      | There is no dependence on engine load or speed.

== system lib_fuel_cell2/fuel converter <fc> net model/Subsystem/Subsystem/fuel use and EO emis Fuel Cell/fc temp correct/fc temp correct Constant Correction Factors (Equation Based)/Block NOTES ==
  note: This block determines actual fuel use and engine-out emissions
      | given the fully hot values and the engine coolant temperature.
      | The correlations used here were developed at NREL using
      | Hot and Cold Engine data collected
      | at Oak Ridge National Laboratory.
